simulink model "positionloop"  (R2024a)
settings: Solver=FixedStepAuto  StartTime=0.0  StopTime=5  FixedStep=1e-4  RelTol=1e-3
undefined symbols (not defined in the file): curr_d_ki, curr_d_kp, curr_q_ki, curr_q_kp, Ke, Kt, Pn, spd_ki, spd_kp, Udc
libraries: slpidlib x12, simulink x7, mcbplantlib x2, autolibpmsmexterior x2
(part 1 of 2)
settings Model: DataDictionary=positionloop.sldd  VariantFading=off  Creator=Administrator  LastModifiedBy=WuHongrui
settings OptimizationCC: DefaultParameterBehavior=Inlined  UseDivisionForNetSlopeComputation=on  GainParamInheritBuiltInType=on  UseFloatMulNetSlope=on  InlineInvariantSignals=on  PassReuseOutputArgsAs=Individual arguments  ZeroExternalMemoryAtStartup=off  ZeroInternalMemoryAtStartup=off  NoFixptDivByZeroProtection=on  EfficientFloat2IntCast=on  LifeSpan=1  OptimizeBlockOrder=speed  DifferentSizesBufferReuse=on  EfficientTunableParamExpr=on
settings DebuggingCC: ParameterTunabilityLossMsg=error  UnconnectedInputMsg=warning  UnconnectedOutputMsg=warning  UnconnectedLineMsg=warning
settings HardwareCC: ProdBitPerPointer=32  ProdBitPerSizeT=32  ProdBitPerPtrDiffT=32  ProdLargestAtomicInteger=Long  ProdLargestAtomicFloat=Double  ProdWordSize=32  ProdLongLongMode=on  ProdHWDeviceType=ARM Compatible->ARM Cortex-M
settings ModelReferenceCC: EnableRefExpFcnMdlSchedulingChecks=on
settings SFSimCC: MATLABDynamicMemAlloc=off
settings RTWCC: Description=Embedded Coder  SystemTargetFile=ert.tlc  GenCodeOnly=on  TemplateMakefile=ert_default_tmf  GenerateReport=on  LaunchReport=on  GenerateCodeReplacementReport=on  GPUComputeCapability=3.5  DLArmComputeVersion=19.05
settings CodeAppCC: ForceParamTrailComments=on  IgnoreCustomStorageClasses=off  OperatorAnnotations=on  SimulinkDataObjDesc=on  SFDataObjDesc=on  CustomSymbolStrGlobalVar=rt$N$M  CustomSymbolStrType=$N$M  CustomSymbolStrFcn=$N$M$F  CustomSymbolStrMacro=$N$M  InsertBlockDesc=on
settings ERTTargetCC: TargetLangStandard=C99 (ISO)  CodeReplacementLibrary=ARM Cortex-M  IncludeMdlTerminateFcn=off  CombineSignalStateStructs=on  SuppressErrorStatus=on  SupportAbsoluteTime=off  SupportComplex=off  InlinedParameterPlacement=NonHierarchical  ERTCustomFileTemplate=example_file_process.tlc  ERTFilePackagingFormat=CompactWithDataFile

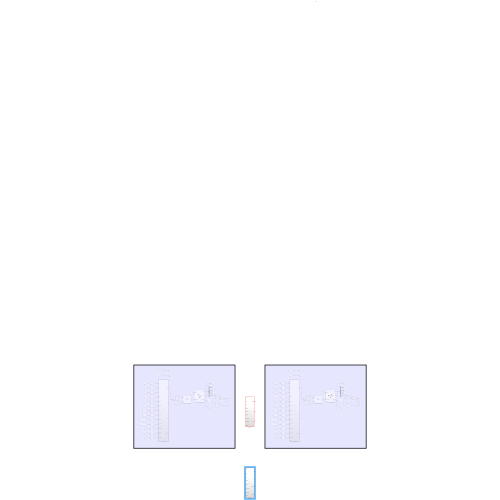
[thumbnail: Simulink's stored preview of the top-level diagram]
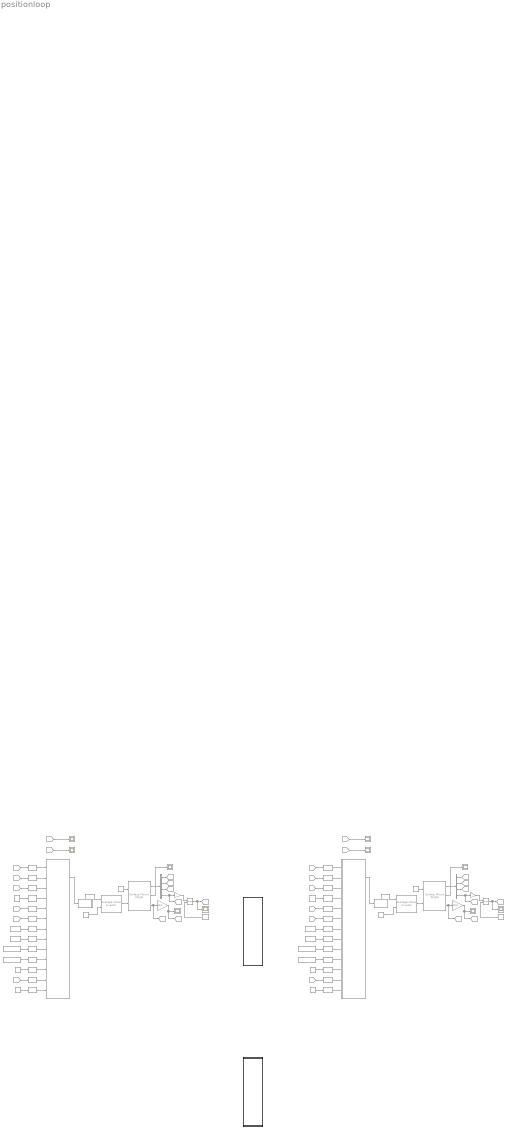
== system positionloop ==
  note: rad
  note: rad/s
  note: rpm
  note: rpm
  note: rad/s
  note: rpm
  note: rpm
  Average-Value Inverter3 : mcbplantlib/Average-Value Inverter  Commented=on
  Average-Value Inverter4 : mcbplantlib/Average-Value Inverter  Commented=on
  Bus Selector3 : BusSelector  Commented=on  OutputSignals=IaStator,IbStator,IcStator,MtrPos
  Bus Selector4 : BusSelector  Commented=on  OutputSignals=IaStator,IbStator,IcStator,MtrPos
  Constant26 : Constant  Commented=on  Value=0
  Constant28 : Constant  Commented=on  Value=0.515264878487547
  Constant34 : Constant  Commented=on  Value=pi/2
  Constant35 : Constant  Commented=on  Value=2*pi  OutDataTypeStr=single
  Constant36 : Constant  Commented=on  Value=0.003389
  Constant37 : Constant  Commented=on  Value=0.00144
  Constant38 : Constant  Commented=on  Value=Udc
  Constant39 : Constant  Commented=on  Value=Udc  OutDataTypeStr=single
  Constant40 : Constant  Commented=on  Value=987.649638453674
  Constant41 : Constant  Commented=on  Value=5
  Constant42 : Constant  Commented=on  Value=0
  Constant43 : Constant  Commented=on  Value=0.515264878487547
  Constant44 : Constant  Commented=on  Value=pi/2
  Constant45 : Constant  Commented=on  Value=2*pi  OutDataTypeStr=single
  Constant46 : Constant  Commented=on  Value=0.003389
  Constant47 : Constant  Commented=on  Value=0.00144
  Constant48 : Constant  Commented=on  Value=Udc
  Constant49 : Constant  Commented=on  Value=Udc  OutDataTypeStr=single
  Constant50 : Constant  Commented=on  Value=987.649638453674
  Constant51 : Constant  Commented=on  Value=5
  Data Type Conversion{35..60} (26 alike) : DataTypeConversion  Commented=on  OutDataTypeStr=single  SaturateOnIntegerOverflow=off  RndMeth=Floor
  From21 : From  Commented=on  GotoTag=ib
  From22 : From  Commented=on  GotoTag=ic
  From23 : From  Commented=on  GotoTag=W
  From24 : From  Commented=on  GotoTag=ia
  From25 : From  Commented=on  GotoTag=theta_e  TagVisibility=global
  From26 : From  Commented=on  GotoTag=Wrpm
  From{27..28,35..36} (4 alike) : From  Commented=on  GotoTag=theta  TagVisibility=global
  From29 : From  Commented=on  GotoTag=ib
  From30 : From  Commented=on  GotoTag=ic
  From31 : From  Commented=on  GotoTag=W
  From32 : From  Commented=on  GotoTag=ia
  From33 : From  Commented=on  GotoTag=theta_e  TagVisibility=global
  From34 : From  Commented=on  GotoTag=Wrpm
  Gain10 : Gain  Commented=on  Gain=Pn  OutDataTypeStr=single
  Gain7 : Gain  Commented=on  Gain=30/pi  OutDataTypeStr=single
  Gain8 : Gain  Commented=on  Gain=Pn  OutDataTypeStr=single
  Gain9 : Gain  Commented=on  Gain=30/pi  OutDataTypeStr=single
  Goto21 : Goto  Commented=on  GotoTag=ib
  Goto22 : Goto  Commented=on  GotoTag=ic
  Goto23 : Goto  Commented=on  GotoTag=theta_e  TagVisibility=global
  Goto24 : Goto  Commented=on  GotoTag=Wrpm
  Goto25 : Goto  Commented=on  GotoTag=W
  Goto26 : Goto  Commented=on  GotoTag=theta  TagVisibility=global
  Goto27 : Goto  Commented=on  GotoTag=ia
  Goto28 : Goto  Commented=on  GotoTag=ib
  Goto29 : Goto  Commented=on  GotoTag=ic
  Goto30 : Goto  Commented=on  GotoTag=theta_e  TagVisibility=global
  Goto31 : Goto  Commented=on  GotoTag=Wrpm
  Goto32 : Goto  Commented=on  GotoTag=W
  Goto33 : Goto  Commented=on  GotoTag=theta  TagVisibility=global
  Goto34 : Goto  Commented=on  GotoTag=ia
  Mod4 : Math  Commented=on  Operator=mod  OutputSignalType=real
  Mod5 : Math  Commented=on  Operator=mod  OutputSignalType=real
  Scope{17..26} (10 alike) : Scope  Commented=on
  Subsystem3 : Subsystem  Commented=on
      settings: PortSchema="{\"entries\":[{\"content\":{\"sides\":[{\"content\":{\"connectorIds\":[\"In1\"]},\"type\":\"ConnectorPlacement.EquallySpacedRectSide\",\"uuid\":\"8ccc51de-fa2a-4900-80a3-4cdf9aa76f01\"},{\"content\":{\"connectorIds\":[],\"side\":\"RIGHT\"},\"type\":\"ConnectorPlacement.EquallySpacedRectSide\",\"uuid\":\"32c06e0d-3f1d-4948-af96-e310e54308a0\"},{\"content\":{\"connectorIds\":[\"Out1\"],\"side\":\"TOP\"},\"type\":\"ConnectorPlacement.EquallySpacedRectSide\",\"uuid\":\"a9066067-2c54-42a8-b4d7-fb86ac71b860\"}]},\"type\":\"ConnectorPlacement.EquallySpacedConnector\",\"uuid\":\"e4576975-acad-4e16-822f-2c2e7f23d7a7\"}],\"packageUris\":[\"http://schema.mathworks.com/mf0/Connector/R2020b\"],\"version\":\"1.0\"}"
  Subsystem4 : Subsystem  Commented=on
      settings: PortSchema="{\"entries\":[{\"content\":{\"sides\":[{\"content\":{\"connectorIds\":[\"In1\"]},\"type\":\"ConnectorPlacement.EquallySpacedRectSide\",\"uuid\":\"8ccc51de-fa2a-4900-80a3-4cdf9aa76f01\"},{\"content\":{\"connectorIds\":[],\"side\":\"RIGHT\"},\"type\":\"ConnectorPlacement.EquallySpacedRectSide\",\"uuid\":\"32c06e0d-3f1d-4948-af96-e310e54308a0\"},{\"content\":{\"connectorIds\":[\"Out1\"],\"side\":\"TOP\"},\"type\":\"ConnectorPlacement.EquallySpacedRectSide\",\"uuid\":\"a9066067-2c54-42a8-b4d7-fb86ac71b860\"}]},\"type\":\"ConnectorPlacement.EquallySpacedConnector\",\"uuid\":\"e4576975-acad-4e16-822f-2c2e7f23d7a7\"}],\"packageUris\":[\"http://schema.mathworks.com/mf0/Connector/R2020b\"],\"version\":\"1.0\"}"
  Surface Mount PMSM3 : autolibpmsmexterior/Surface Mount PMSM  Commented=on  port_config=Torque  sim_type=Discrete  Ts=1e-4  P=Pn  Rs=Rs  Ldq_=L  KConstText=Torque constant (Kt):  lambda_pm=flux  Ke=0.0059268  Kt=Kt  mechanical=[0.096e-4, 2e-5, 0]  idq0=[0 0]  theta_init=0  omega_init=0  KConst=Kt  lambda_pm_calc=0.011  RefBlkName='autolibpmsmexterior/Surface Mount PMSM'  aMode=5  Ldq="[0.0017      0.0017]"
  Surface Mount PMSM4 : autolibpmsmexterior/Surface Mount PMSM  Commented=on  port_config=Torque  sim_type=Discrete  Ts=1e-4  P=Pn  Rs=Rs  Ldq_=L  KConstText=Torque constant (Kt):  lambda_pm=flux  Ke=0.0059268  Kt=Kt  mechanical=[0.096e-4, 2e-5, 0]  idq0=[0 0]  theta_init=0  omega_init=0  KConst=Kt  lambda_pm_calc=0.011  RefBlkName='autolibpmsmexterior/Surface Mount PMSM'  aMode=5  Ldq="[0.0017      0.0017]"
  currloop : Subsystem  TreatAsAtomicUnit=on
  currloop1 : Subsystem  TreatAsAtomicUnit=on
  triloop_feedforward : Subsystem  Commented=on  TreatAsAtomicUnit=on
  triloop_tune : Subsystem  Commented=on  TreatAsAtomicUnit=on
  wires:
  Surface Mount PMSM3/3 -> Gain7/1, Goto25/1
  Data Type Conversion42/1 -> triloop_tune/6(SpeedFd)
  triloop_tune/1(tABC) -> Subsystem3/1(DutyIn)
  Data Type Conversion36/1 -> triloop_tune/2(ib)
  Surface Mount PMSM3/1 -> Bus Selector3/1
  Bus Selector3/3 -> Goto22/1  "<IcStator>"
  Bus Selector3/4 -> Goto26/1, Gain8/1  "<MtrPos>"
  Subsystem3/1(DutyOut) -> Average-Value Inverter3/1
  Average-Value Inverter3/1 -> Surface Mount PMSM3/2
  From24/1 -> Data Type Conversion35/1
  Bus Selector3/2 -> Goto21/1  "<IbStator>"
  Constant35/1 -> Mod4/2
  Constant38/1 -> Average-Value Inverter3/2
  Mod4/1 -> Scope19/1, Goto23/1
  From22/1 -> Data Type Conversion38/1
  Bus Selector3/1 -> Goto27/1  "<IaStator>"
  Constant36/1 -> Data Type Conversion43/1
  From21/1 -> Data Type Conversion36/1
  Constant28/1 -> Data Type Conversion45/1
  Data Type Conversion44/1 -> triloop_tune/8(I_speed)
  From25/1 -> Data Type Conversion41/1
  Data Type Conversion45/1 -> triloop_tune/9(P_current)
  From23/1 -> Data Type Conversion42/1
  Data Type Conversion43/1 -> triloop_tune/7(P_speed)
  Data Type Conversion41/1 -> triloop_tune/5(theta_e)
  Gain8/1 -> Mod4/1
  Data Type Conversion39/1 -> triloop_tune/4(VBUS)
  Surface Mount PMSM3/2 -> Scope18/1  "Iab_fb"
  Data Type Conversion35/1 -> triloop_tune/1(ia)
  From26/1 -> Scope20/1
  Gain7/1 -> Scope17/1, Goto24/1
  Constant26/1 -> Surface Mount PMSM3/1
  Constant39/1 -> Data Type Conversion39/1
  Data Type Conversion38/1 -> triloop_tune/3(ic)
  Data Type Conversion37/1 -> triloop_tune/10(I_current)
  Constant40/1 -> Data Type Conversion37/1
  Constant37/1 -> Data Type Conversion44/1
  Data Type Conversion47/1 -> triloop_tune/13(P_position)
  Data Type Conversion46/1 -> triloop_tune/12(PositionFd)
  Data Type Conversion40/1 -> triloop_tune/11(PositionRef)
  Constant34/1 -> Data Type Conversion40/1
  From27/1 -> Data Type Conversion46/1
  Constant41/1 -> Data Type Conversion47/1
  From28/1 -> Scope21/1
  Data Type Conversion53/1 -> triloop_feedforward/11(PositionRef)
  Constant51/1 -> Data Type Conversion60/1
  Constant42/1 -> Surface Mount PMSM4/1
  From34/1 -> Scope25/1
  From31/1 -> Data Type Conversion55/1
  Data Type Conversion60/1 -> triloop_feedforward/13(P_position)
  Data Type Conversion57/1 -> triloop_feedforward/8(I_speed)
  Data Type Conversion58/1 -> triloop_feedforward/9(P_current)
  Data Type Conversion54/1 -> triloop_feedforward/5(theta_e)
  Data Type Conversion48/1 -> triloop_feedforward/1(ia)
  Surface Mount PMSM4/2 -> Scope23/1  "Iab_fb"
  Gain10/1 -> Mod5/1
  Data Type Conversion59/1 -> triloop_feedforward/12(PositionFd)
  Constant43/1 -> Data Type Conversion58/1
  Data Type Conversion52/1 -> triloop_feedforward/4(VBUS)
  Data Type Conversion56/1 -> triloop_feedforward/7(P_speed)
  From30/1 -> Data Type Conversion51/1
  From29/1 -> Data Type Conversion49/1
  Gain9/1 -> Scope22/1, Goto31/1
  Constant48/1 -> Average-Value Inverter4/2
  Constant46/1 -> Data Type Conversion56/1
  Mod5/1 -> Scope24/1, Goto30/1
  Bus Selector4/3 -> Goto29/1  "<IcStator>"
  Bus Selector4/2 -> Goto28/1  "<IbStator>"
  Data Type Conversion49/1 -> triloop_feedforward/2(ib)
  Bus Selector4/4 -> Goto33/1, Gain10/1  "<MtrPos>"
  Constant45/1 -> Mod5/2
  Average-Value Inverter4/1 -> Surface Mount PMSM4/2
  Surface Mount PMSM4/1 -> Bus Selector4/1
  Subsystem4/1(DutyOut) -> Average-Value Inverter4/1
  Surface Mount PMSM4/3 -> Gain9/1, Goto32/1
  From33/1 -> Data Type Conversion54/1
  From32/1 -> Data Type Conversion48/1
  triloop_feedforward/1(tABC) -> Subsystem4/1(DutyIn)
  Data Type Conversion55/1 -> triloop_feedforward/6(SpeedFd)
  Data Type Conversion51/1 -> triloop_feedforward/3(ic)
  Constant50/1 -> Data Type Conversion50/1
  Constant49/1 -> Data Type Conversion52/1
  Constant47/1 -> Data Type Conversion57/1
  Constant44/1 -> Data Type Conversion53/1
  Data Type Conversion50/1 -> triloop_feedforward/10(I_current)
  Bus Selector4/1 -> Goto34/1  "<IaStator>"
  From35/1 -> Data Type Conversion59/1
  From36/1 -> Scope26/1

== system positionloop/Subsystem3 ==
  DutyIn : Inport
  Constant : Constant  Value=0.5  SampleTime=-1
  Gain : Gain  Gain=1/8000  ParamDataTypeStr=single
  Gain1 : Gain  Gain=-1
  Sum : Sum  Inputs=|+-
  Sum1 : Sum  Inputs=|++
  DutyOut : Outport
  wires:
  Sum/1 -> Gain1/1
  Constant/1 -> Sum1/2, Sum/2
  DutyIn/1 -> Gain/1
  Gain1/1 -> Sum1/1
  Sum1/1 -> DutyOut/1
  Gain/1 -> Sum/1

== system positionloop/Subsystem4 ==
  DutyIn : Inport
  Constant : Constant  Value=0.5  SampleTime=-1
  Gain : Gain  Gain=1/8000  ParamDataTypeStr=single
  Gain1 : Gain  Gain=-1
  Sum : Sum  Inputs=|+-
  Sum1 : Sum  Inputs=|++
  DutyOut : Outport
  wires:
  Sum/1 -> Gain1/1
  Constant/1 -> Sum1/2, Sum/2
  DutyIn/1 -> Gain/1
  Gain1/1 -> Sum1/1
  Sum1/1 -> DutyOut/1
  Gain/1 -> Sum/1

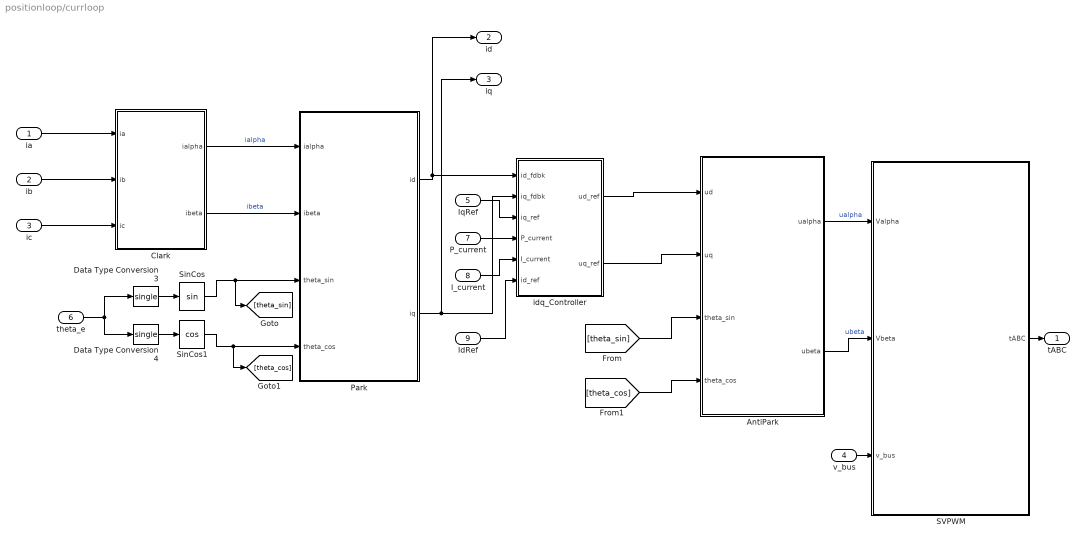
== system positionloop/currloop ==
  ia : Inport
  ib : Inport  Port=2
  ic : Inport  Port=3
  v_bus : Inport  Port=4
  IqRef : Inport  Port=5
  theta_e : Inport  Port=6
  P_current : Inport  Port=7
  I_current : Inport  Port=8
  IdRef : Inport  Port=9
  AntiPark : Subsystem
  Clark : Subsystem
  Data Type Conversion3 : DataTypeConversion  OutDataTypeStr=single  SaturateOnIntegerOverflow=off  RndMeth=Floor
  Data Type Conversion4 : DataTypeConversion  OutDataTypeStr=single  SaturateOnIntegerOverflow=off  RndMeth=Floor
  Park : Subsystem
  SVPWM : Subsystem  TreatAsAtomicUnit=on
  SinCos : Trigonometry
  SinCos1 : Trigonometry  Operator=cos
  idq_Controller : Subsystem
  tABC : Outport
  id : Outport  Port=2
  iq : Outport  Port=3
  wires:
  Data Type Conversion4/1 -> SinCos1/1
  Data Type Conversion3/1 -> SinCos/1
  AntiPark/2(ubeta) -> SVPWM/2(Vbeta)  "ubeta"
  AntiPark/1(ualpha) -> SVPWM/1(Valpha)  "ualpha"
  [theta_cos] -> AntiPark/4(theta_cos)
  [theta_sin] -> AntiPark/3(theta_sin)
  SinCos/1 -> Park/3(theta_sin), [theta_sin]
  theta_e/1 -> Data Type Conversion3/1, Data Type Conversion4/1
  SinCos1/1 -> Park/4(theta_cos), [theta_cos]
  v_bus/1 -> SVPWM/3(v_bus)
  SVPWM/1(tABC) -> tABC/1
  ib/1 -> Clark/2(ib)
  ia/1 -> Clark/1(ia)
  ic/1 -> Clark/3(ic)
  Clark/1(ialpha) -> Park/1(ialpha)  "ialpha"
  Clark/2(ibeta) -> Park/2(ibeta)  "ibeta"
  idq_Controller/1(ud_ref) -> AntiPark/1(ud)
  idq_Controller/2(uq_ref) -> AntiPark/2(uq)
  Park/1(id) -> id/1, idq_Controller/1(id_fdbk)
  Park/2(iq) -> iq/1, idq_Controller/2(iq_fdbk)
  IqRef/1 -> idq_Controller/3(iq_ref)
  I_current/1 -> idq_Controller/5(I_current)
  P_current/1 -> idq_Controller/4(P_current)
  IdRef/1 -> idq_Controller/6(id_ref)

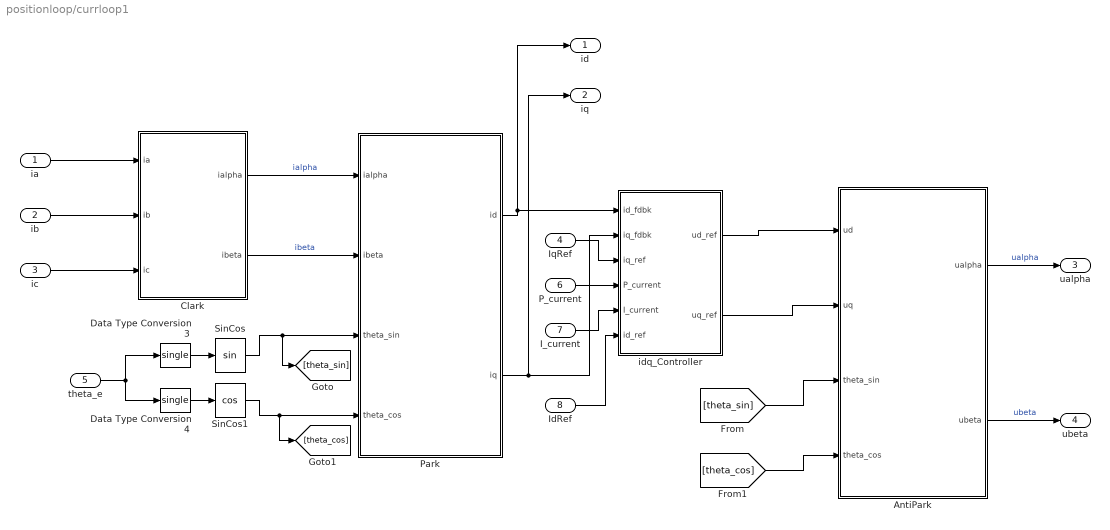
== system positionloop/currloop1 ==
  ia : Inport
  ib : Inport  Port=2
  ic : Inport  Port=3
  IqRef : Inport  Port=4
  theta_e : Inport  Port=5
  P_current : Inport  Port=6
  I_current : Inport  Port=7
  IdRef : Inport  Port=8
  AntiPark : Subsystem
  Clark : Subsystem
  Data Type Conversion3 : DataTypeConversion  OutDataTypeStr=single  SaturateOnIntegerOverflow=off  RndMeth=Floor
  Data Type Conversion4 : DataTypeConversion  OutDataTypeStr=single  SaturateOnIntegerOverflow=off  RndMeth=Floor
  Park : Subsystem
  SinCos : Trigonometry
  SinCos1 : Trigonometry  Operator=cos
  idq_Controller : Subsystem
  id : Outport
  iq : Outport  Port=2
  ualpha : Outport  Port=3
  ubeta : Outport  Port=4
  wires:
  Data Type Conversion4/1 -> SinCos1/1
  Data Type Conversion3/1 -> SinCos/1
  [theta_cos] -> AntiPark/4(theta_cos)
  [theta_sin] -> AntiPark/3(theta_sin)
  SinCos/1 -> Park/3(theta_sin), [theta_sin]
  theta_e/1 -> Data Type Conversion3/1, Data Type Conversion4/1
  SinCos1/1 -> Park/4(theta_cos), [theta_cos]
  ib/1 -> Clark/2(ib)
  ia/1 -> Clark/1(ia)
  ic/1 -> Clark/3(ic)
  Clark/1(ialpha) -> Park/1(ialpha)  "ialpha"
  Clark/2(ibeta) -> Park/2(ibeta)  "ibeta"
  idq_Controller/1(ud_ref) -> AntiPark/1(ud)
  idq_Controller/2(uq_ref) -> AntiPark/2(uq)
  Park/1(id) -> id/1, idq_Controller/1(id_fdbk)
  Park/2(iq) -> iq/1, idq_Controller/2(iq_fdbk)
  IqRef/1 -> idq_Controller/3(iq_ref)
  I_current/1 -> idq_Controller/5(I_current)
  P_current/1 -> idq_Controller/4(P_current)
  IdRef/1 -> idq_Controller/6(id_ref)
  AntiPark/1(ualpha) -> ualpha/1  "ualpha"
  AntiPark/2(ubeta) -> ubeta/1  "ubeta"

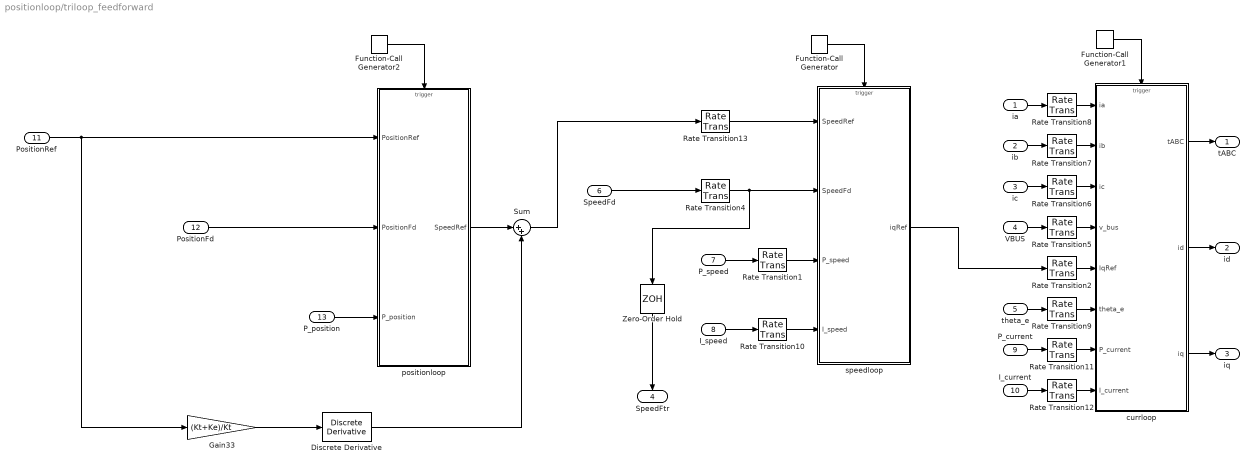
== system positionloop/triloop_feedforward ==
  ia : Inport
  ib : Inport  Port=2
  ic : Inport  Port=3
  VBUS : Inport  Port=4
  theta_e : Inport  Port=5
  SpeedFd : Inport  Port=6
  P_speed : Inport  Port=7
  I_speed : Inport  Port=8
  P_current : Inport  Port=9
  I_current : Inport  Port=10
  PositionRef : Inport  Port=11
  PositionFd : Inport  Port=12
  P_position : Inport  Port=13
  Discrete Derivative : simulink/Discrete/Discrete Derivative  gainval=0.35  ICPrevScaledInput=0.0  OutMin=[]  OutMax=[]  OutDataType=fixdt(1, 16)  OutScaling=2^-10  DoSatur=off
  Function-Call Generator : simulink/Ports & Subsystems/Function-Call Generator  sample_time=1e-3  numberOfIterations=1  DisallowWideOutput=off
  Function-Call Generator1 : simulink/Ports & Subsystems/Function-Call Generator  sample_time=1e-4  numberOfIterations=1  DisallowWideOutput=off
  Function-Call Generator2 : simulink/Ports & Subsystems/Function-Call Generator  sample_time=1e-2  numberOfIterations=1  DisallowWideOutput=off
  Gain33 : Gain  Gain=(Kt+Ke)/Kt
  Rate Transition{1..2,4..13} (12 alike) : RateTransition
  Sum : Sum  Inputs=|++
  Zero-Order Hold : ZeroOrderHold  SampleTime=-1
  currloop : Subsystem  TreatAsAtomicUnit=on
  positionloop : Subsystem
  speedloop : Subsystem
  tABC : Outport
  id : Outport  Port=2
  iq : Outport  Port=3
  SpeedFtr : Outport  Port=4
  wires:
  currloop/1(tABC) -> tABC/1
  VBUS/1 -> Rate Transition5/1
  ib/1 -> Rate Transition7/1
  ia/1 -> Rate Transition8/1
  ic/1 -> Rate Transition6/1
  Function-Call Generator/1 -> speedloop/Trigger
  Rate Transition13/1 -> speedloop/1(SpeedRef)
  theta_e/1 -> Rate Transition9/1
  Rate Transition2/1 -> currloop/5(IqRef)
  Rate Transition5/1 -> currloop/4(v_bus)
  Rate Transition6/1 -> currloop/3(ic)
  Rate Transition7/1 -> currloop/2(ib)
  Rate Transition8/1 -> currloop/1(ia)
  Rate Transition9/1 -> currloop/6(theta_e)
  Rate Transition4/1 -> speedloop/2(SpeedFd), Zero-Order Hold/1
  SpeedFd/1 -> Rate Transition4/1
  Function-Call Generator1/1 -> currloop/Trigger
  P_speed/1 -> Rate Transition1/1
  I_speed/1 -> Rate Transition10/1
  P_current/1 -> Rate Transition11/1
  I_current/1 -> Rate Transition12/1
  speedloop/1(iqRef) -> Rate Transition2/1
  Rate Transition1/1 -> speedloop/3(P_speed)
  Rate Transition10/1 -> speedloop/4(I_speed)
  Rate Transition11/1 -> currloop/7(P_current)
  Rate Transition12/1 -> currloop/8(I_current)
  currloop/3(iq) -> iq/1
  currloop/2(id) -> id/1
  Zero-Order Hold/1 -> SpeedFtr/1
  PositionFd/1 -> positionloop/2(PositionFd)
  P_position/1 -> positionloop/3(P_position)
  Function-Call Generator2/1 -> positionloop/Trigger
  Gain33/1 -> Discrete Derivative/1
  Sum/1 -> Rate Transition13/1
  positionloop/1(SpeedRef) -> Sum/1
  PositionRef/1 -> Gain33/1, positionloop/1(PositionRef)
  Discrete Derivative/1 -> Sum/2

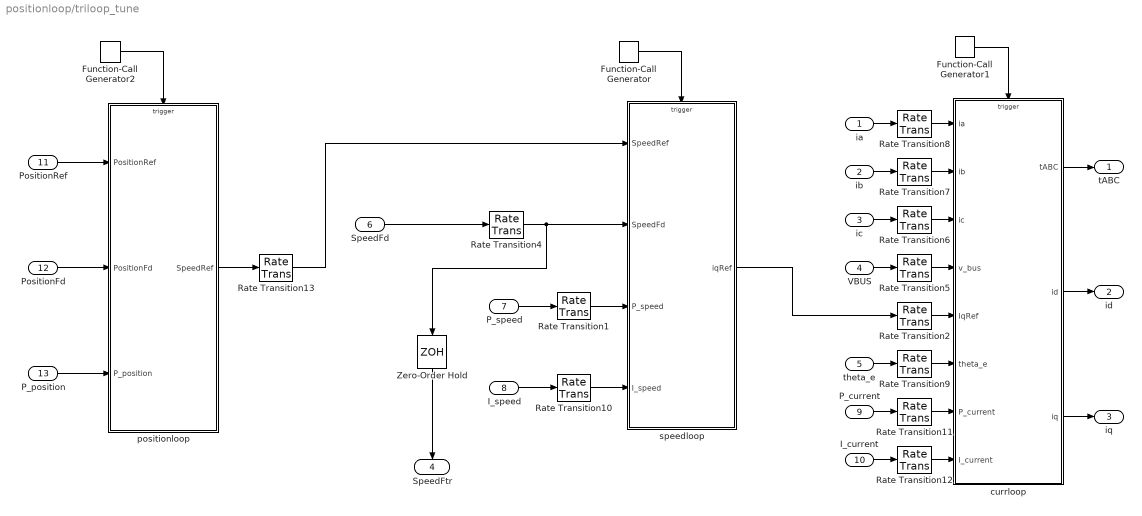
== system positionloop/triloop_tune ==
  ia : Inport
  ib : Inport  Port=2
  ic : Inport  Port=3
  VBUS : Inport  Port=4
  theta_e : Inport  Port=5
  SpeedFd : Inport  Port=6
  P_speed : Inport  Port=7
  I_speed : Inport  Port=8
  P_current : Inport  Port=9
  I_current : Inport  Port=10
  PositionRef : Inport  Port=11
  PositionFd : Inport  Port=12
  P_position : Inport  Port=13
  Function-Call Generator : simulink/Ports & Subsystems/Function-Call Generator  sample_time=1e-3  numberOfIterations=1  DisallowWideOutput=off
  Function-Call Generator1 : simulink/Ports & Subsystems/Function-Call Generator  sample_time=1e-4  numberOfIterations=1  DisallowWideOutput=off
  Function-Call Generator2 : simulink/Ports & Subsystems/Function-Call Generator  sample_time=1e-3  numberOfIterations=1  DisallowWideOutput=off
  Rate Transition{1..2,4..13} (12 alike) : RateTransition
  Zero-Order Hold : ZeroOrderHold  SampleTime=-1
  currloop : Subsystem  TreatAsAtomicUnit=on
  positionloop : Subsystem
  speedloop : Subsystem
  tABC : Outport
  id : Outport  Port=2
  iq : Outport  Port=3
  SpeedFtr : Outport  Port=4
  wires:
  currloop/1(tABC) -> tABC/1
  VBUS/1 -> Rate Transition5/1
  ib/1 -> Rate Transition7/1
  ia/1 -> Rate Transition8/1
  ic/1 -> Rate Transition6/1
  Function-Call Generator/1 -> speedloop/Trigger
  Rate Transition13/1 -> speedloop/1(SpeedRef)
  theta_e/1 -> Rate Transition9/1
  Rate Transition2/1 -> currloop/5(IqRef)
  Rate Transition5/1 -> currloop/4(v_bus)
  Rate Transition6/1 -> currloop/3(ic)
  Rate Transition7/1 -> currloop/2(ib)
  Rate Transition8/1 -> currloop/1(ia)
  Rate Transition9/1 -> currloop/6(theta_e)
  Rate Transition4/1 -> speedloop/2(SpeedFd), Zero-Order Hold/1
  SpeedFd/1 -> Rate Transition4/1
  Function-Call Generator1/1 -> currloop/Trigger
  P_speed/1 -> Rate Transition1/1
  I_speed/1 -> Rate Transition10/1
  P_current/1 -> Rate Transition11/1
  I_current/1 -> Rate Transition12/1
  speedloop/1(iqRef) -> Rate Transition2/1
  Rate Transition1/1 -> speedloop/3(P_speed)
  Rate Transition10/1 -> speedloop/4(I_speed)
  Rate Transition11/1 -> currloop/7(P_current)
  Rate Transition12/1 -> currloop/8(I_current)
  currloop/3(iq) -> iq/1
  currloop/2(id) -> id/1
  Zero-Order Hold/1 -> SpeedFtr/1
  positionloop/1(SpeedRef) -> Rate Transition13/1
  PositionRef/1 -> positionloop/1(PositionRef)
  PositionFd/1 -> positionloop/2(PositionFd)
  P_position/1 -> positionloop/3(P_position)
  Function-Call Generator2/1 -> positionloop/Trigger

== system positionloop/currloop/AntiPark ==
  note: Valpha = ud*cos(theta) - uq*sin(theta);
      | Vbeta = ud*sin(theta) + uq*cos(theta);
  ud : Inport
  uq : Inport  Port=2
  theta_sin : Inport  Port=3
  theta_cos : Inport  Port=4
  Add : Sum  Inputs=+-
  Add1 : Sum
  Product{,1..3} (4 alike) : Product
  ualpha : Outport  OutDataTypeStr=single
  ubeta : Outport  Port=2  OutDataTypeStr=single
  wires:
  Product2/1 -> Add1/1
  Product/1 -> Add/1
  Add/1 -> ualpha/1
  Product3/1 -> Add1/2
  ud/1 -> Product/1, Product2/1
  theta_sin/1 -> Product1/2, Product2/2
  theta_cos/1 -> Product3/2, Product/2
  uq/1 -> Product1/1, Product3/1
  Product1/1 -> Add/2
  Add1/1 -> ubeta/1

== system positionloop/currloop/Clark ==
  note: ialpha = ia*2/3-(ib+ic)/3;
      | ibeta = (ib-ic)*sqrt(3)/3;
  ia : Inport  OutDataTypeStr=single
  ib : Inport  Port=2  OutDataTypeStr=single
  ic : Inport  Port=3  OutDataTypeStr=single
  Add : Sum  OutDataTypeStr=single  AccumDataTypeStr=single
  Add1 : Sum  Inputs=+-  OutDataTypeStr=single  AccumDataTypeStr=single
  Add2 : Sum  Inputs=+-  OutDataTypeStr=single  AccumDataTypeStr=single
  Gain : Gain  Gain=2/3  ParamDataTypeStr=single
  Gain1 : Gain  Gain=1/3  ParamDataTypeStr=single
  Gain2 : Gain  Gain=sqrt(3)/3  ParamDataTypeStr=single
  ialpha : Outport  OutDataTypeStr=single
  ibeta : Outport  Port=2  OutDataTypeStr=single
  wires:
  Add1/1 -> ialpha/1
  ia/1 -> Gain/1
  Gain2/1 -> ibeta/1
  ib/1 -> Add/1, Add2/1
  Gain/1 -> Add1/1
  Add2/1 -> Gain2/1
  Add/1 -> Gain1/1
  ic/1 -> Add/2, Add2/2
  Gain1/1 -> Add1/2

== system positionloop/currloop/Park ==
  note: id = ialpha*cos(theta)+ibeta*sin(theta);
      | iq = -ialpha*sin(theta)+ibeta*cos(theta);
  ialpha : Inport  OutDataTypeStr=single
  ibeta : Inport  Port=2  OutDataTypeStr=single
  theta_sin : Inport  Port=3  OutDataTypeStr=single
  theta_cos : Inport  Port=4  OutDataTypeStr=single
  Add : Sum  OutDataTypeStr=single  AccumDataTypeStr=single
  Add1 : Sum  Inputs=-+  OutDataTypeStr=single  AccumDataTypeStr=single
  Product{,1..3} (4 alike) : Product  OutDataTypeStr=single
  id : Outport  OutDataTypeStr=single
  iq : Outport  Port=2  OutDataTypeStr=single
  wires:
  theta_cos/1 -> Product/2, Product3/2
  ibeta/1 -> Product1/1, Product3/1
  Product1/1 -> Add/2
  Add1/1 -> iq/1
  Add/1 -> id/1
  Product3/1 -> Add1/2
  ialpha/1 -> Product/1, Product2/1
  Product2/1 -> Add1/1
  Product/1 -> Add/1
  theta_sin/1 -> Product1/2, Product2/2

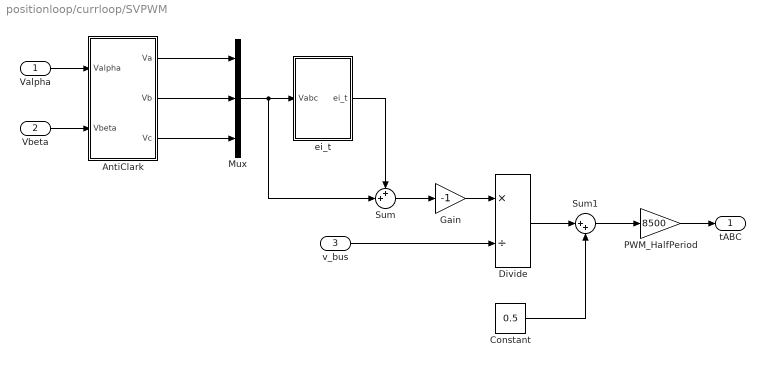
== system positionloop/currloop/SVPWM ==
  Valpha : Inport  OutDataTypeStr=single
  Vbeta : Inport  Port=2  OutDataTypeStr=single
  v_bus : Inport  Port=3  OutDataTypeStr=single
  AntiClark : Subsystem
  Constant : Constant  Value=0.5  OutDataTypeStr=single
  Divide : Product  Inputs=*/  OutDataTypeStr=single
  Gain : Gain  Gain=-1  OutDataTypeStr=single
  Mux : Mux  Inputs=3
  PWM_HalfPeriod : Gain  Gain=8500  OutDataTypeStr=single
  Sum : Sum  Inputs=++|  OutDataTypeStr=single
  Sum1 : Sum  Inputs=|++  OutDataTypeStr=single
  ei_t : Subsystem
  tABC : Outport  OutDataTypeStr=single
  wires:
  Gain/1 -> Divide/1
  v_bus/1 -> Divide/2
  PWM_HalfPeriod/1 -> tABC/1
  Sum1/1 -> PWM_HalfPeriod/1
  Constant/1 -> Sum1/2
  Divide/1 -> Sum1/1
  Mux/1 -> ei_t/1(Vabc), Sum/2
  Sum/1 -> Gain/1
  AntiClark/3(Vc) -> Mux/3
  AntiClark/2(Vb) -> Mux/2
  AntiClark/1(Va) -> Mux/1
  ei_t/1(ei_t) -> Sum/1
  Vbeta/1 -> AntiClark/2(Vbeta)
  Valpha/1 -> AntiClark/1(Valpha)

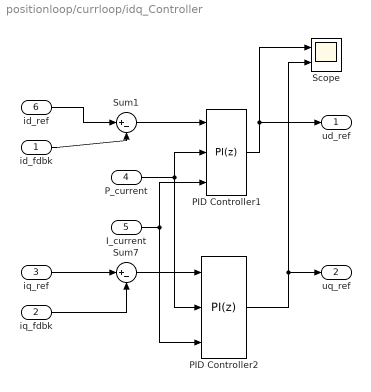
== system positionloop/currloop/idq_Controller ==
  id_fdbk : Inport  OutDataTypeStr=single
  iq_fdbk : Inport  Port=2  OutDataTypeStr=single
  iq_ref : Inport  Port=3  OutDataTypeStr=single
  P_current : Inport  Port=4  OutDataTypeStr=single
  I_current : Inport  Port=5  OutDataTypeStr=single
  id_ref : Inport  Port=6  OutDataTypeStr=single
  PID Controller1 : slpidlib/PID Controller  Controller=PI  Form=Parallel  TimeDomain=Discrete-time  UseExternalTs=off  SampleTime=-1  IntegratorMethod=Forward Euler  FilterMethod=Forward Euler  ControllerParametersSource=external  P=curr_d_kp  I=curr_d_ki  UseKiTs=off  D=0  UseExternalDerivativeSource=off  N=100  UseFilter=on  TunerSelectOption=Transfer Function Based (PID Tuner App)  InitialConditionSource=internal  InitialConditionForIntegrator=0  InitialConditionForFilter=0  DifferentiatorICPrevScaledInput=0  ExternalReset=none  TrackingMode=off  Kt=1  LimitOutput=on  SatLimitsSource=internal  UpperSaturationLimit=48*0.9/sqrt(3)  LowerSaturationLimit=-48*0.9/sqrt(3)  LinearizeAsGain=on  AntiWindupMode=clamping  Kb=1  LimitIntegrator=off  UpperIntegratorSaturationLimit=inf  LowerIntegratorSaturationLimit=-inf  PGainOutDataTypeStr=single  PProdOutDataTypeStr=single  POutMin=[]  POutMax=[]  IGainOutDataTypeStr=int16  IProdOutDataTypeStr=int16  IOutMin=[]  IOutMax=[]  DOutMin=[]  DOutMax=[]  NOutMin=[]  NOutMax=[]  SumOutDataTypeStr=single  SumOutMin=[]  SumOutMax=[]  SaturationOutDataTypeStr=single  SaturationOutMin=[]  SaturationOutMax=[]  PParamMin=[]  PParamMax=[]  IParamMin=[]  IParamMax=[]  DParamMin=[]  DParamMax=[]  NParamMin=[]  NParamMax=[]  KbParamMin=[]  KbParamMax=[]  KtParamMin=[]  KtParamMax=[]  KbOutMin=[]  KbOutMax=[]  KtOutMin=[]  KtOutMax=[]  IntegratorOutMin=[]  IntegratorOutMax=[]  FilterOutMin=[]  FilterOutMax=[]  SumI1OutMin=[]  SumI1OutMax=[]  SumI2OutMin=[]  SumI2OutMax=[]  SumI3OutMin=[]  SumI3OutMax=[]  SumI4OutMin=[]  SumI4OutMax=[]  SumDOutMin=[]  SumDOutMax=[]  DifferentiatorOutMin=[]  DifferentiatorOutMax=[]  FilterDiffOutCoefMin=[]  FilterDiffOutCoefMax=[]  ReciprocalOutMin=[]  ReciprocalOutMax=[]  SumDenOutMin=[]  SumDenOutMax=[]  SumNumOutMin=[]  SumNumOutMax=[]  DivideOutMin=[]  DivideOutMax=[]  UdiffTsProdOutMin=[]  UdiffTsProdOutMax=[]  NTsProdOutMin=[]  NTsProdOutMax=[]  UintegralTsProdOutMin=[]  UintegralTsProdOutMax=[]  UngainTsProdOutMin=[]  UngainTsProdOutMax=[]  ClampingZeroOutDataTypeStr=Inherit: Inherit via back propagation  ClampingZeroOutMin=[]  ClampingZeroOutMax=[]  FilterDenConstantOutDataTypeStr=Inherit: Inherit via back propagation  FilterDenConstantOutMin=[]  FilterDenConstantOutMax=[]  PCopyOutDataTypeStr=Inherit: Inherit via back propagation  PCopyOutMin=[]  PCopyOutMax=[]  NCopyOutDataTypeStr=Inherit: Inherit via back propagation  NCopyOutMin=[]  NCopyOutMax=[]  IntegratorContinuousStateAttributes=''  IntegratorStateMustResolveToSignalObject=off  IntegratorRTWStateStorageClass=Auto  FilterContinuousStateAttributes=''  FilterStateMustResolveToSignalObject=off  FilterRTWStateStorageClass=Auto  ParallelPVariant=ExternalParameters  IdealPVariant=Disabled  IVariant=ExternalParameters  DVariant=Disabled  IntegratorVariant=Discrete  SatVariant=Enabled  AWVariant=DiscClampingParallel  PCopyVariant=Disabled  TRVariant=Disabled  FdbkBlocksVariant=Forward  IdealPFdbkVariant=Disabled  SatFdbkVariant=Disabled  DerivativeFilterVariant=Disabled  NVariant=Disabled  NCopyVariant=Disabled_SignalSpec  FilterICVariant=Disabled  IntegratorICVariant=InternalICs  ExternalResetVariant=Disabled  TRSumVariant=Passthrough  SumFdbkVariant=Disabled  SumVariant=Sum_PI  TsampFilterVariant=InternalTs  TsampNgainVariant=Passthrough  TsampIntegralVariant=Disabled_SignalSpec  ExternalSaturationOutDataTypeStr=Inherit: Same as second input  DerivativeSourceVariant=Disabled
  PID Controller2 : slpidlib/PID Controller  Controller=PI  Form=Parallel  TimeDomain=Discrete-time  UseExternalTs=off  SampleTime=-1  IntegratorMethod=Forward Euler  FilterMethod=Forward Euler  ControllerParametersSource=external  P=curr_q_kp  I=curr_q_ki  UseKiTs=off  D=0  UseExternalDerivativeSource=off  N=100  UseFilter=on  TunerSelectOption=Transfer Function Based (PID Tuner App)  InitialConditionSource=internal  InitialConditionForIntegrator=0  InitialConditionForFilter=0  DifferentiatorICPrevScaledInput=0  ExternalReset=none  TrackingMode=off  Kt=1  LimitOutput=on  SatLimitsSource=internal  UpperSaturationLimit=48*0.9/sqrt(3)  LowerSaturationLimit=-48*0.9/sqrt(3)  LinearizeAsGain=on  AntiWindupMode=clamping  Kb=1  LimitIntegrator=off  UpperIntegratorSaturationLimit=inf  LowerIntegratorSaturationLimit=-inf  PGainOutDataTypeStr=single  PProdOutDataTypeStr=single  POutMin=[]  POutMax=[]  IGainOutDataTypeStr=single  IProdOutDataTypeStr=single  IOutMin=[]  IOutMax=[]  DOutMin=[]  DOutMax=[]  NOutMin=[]  NOutMax=[]  SumOutDataTypeStr=single  SumOutMin=[]  SumOutMax=[]  SaturationOutDataTypeStr=single  SaturationOutMin=[]  SaturationOutMax=[]  PParamMin=[]  PParamMax=[]  IParamMin=[]  IParamMax=[]  DParamMin=[]  DParamMax=[]  NParamMin=[]  NParamMax=[]  KbParamMin=[]  KbParamMax=[]  KtParamMin=[]  KtParamMax=[]  KbOutMin=[]  KbOutMax=[]  KtOutMin=[]  KtOutMax=[]  IntegratorOutMin=[]  IntegratorOutMax=[]  FilterOutMin=[]  FilterOutMax=[]  SumI1OutMin=[]  SumI1OutMax=[]  SumI2OutMin=[]  SumI2OutMax=[]  SumI3OutMin=[]  SumI3OutMax=[]  SumI4OutMin=[]  SumI4OutMax=[]  SumDOutMin=[]  SumDOutMax=[]  DifferentiatorOutMin=[]  DifferentiatorOutMax=[]  FilterDiffOutCoefMin=[]  FilterDiffOutCoefMax=[]  ReciprocalOutMin=[]  ReciprocalOutMax=[]  SumDenOutMin=[]  SumDenOutMax=[]  SumNumOutMin=[]  SumNumOutMax=[]  DivideOutMin=[]  DivideOutMax=[]  UdiffTsProdOutMin=[]  UdiffTsProdOutMax=[]  NTsProdOutMin=[]  NTsProdOutMax=[]  UintegralTsProdOutMin=[]  UintegralTsProdOutMax=[]  UngainTsProdOutMin=[]  UngainTsProdOutMax=[]  ClampingZeroOutDataTypeStr=Inherit: Inherit via back propagation  ClampingZeroOutMin=[]  ClampingZeroOutMax=[]  FilterDenConstantOutDataTypeStr=Inherit: Inherit via back propagation  FilterDenConstantOutMin=[]  FilterDenConstantOutMax=[]  PCopyOutDataTypeStr=Inherit: Inherit via back propagation  PCopyOutMin=[]  PCopyOutMax=[]  NCopyOutDataTypeStr=Inherit: Inherit via back propagation  NCopyOutMin=[]  NCopyOutMax=[]  IntegratorContinuousStateAttributes=''  IntegratorStateMustResolveToSignalObject=off  IntegratorRTWStateStorageClass=Auto  FilterContinuousStateAttributes=''  FilterStateMustResolveToSignalObject=off  FilterRTWStateStorageClass=Auto  ParallelPVariant=ExternalParameters  IdealPVariant=Disabled  IVariant=ExternalParameters  DVariant=Disabled  IntegratorVariant=Discrete  SatVariant=Enabled  AWVariant=DiscClampingParallel  PCopyVariant=Disabled  TRVariant=Disabled  FdbkBlocksVariant=Forward  IdealPFdbkVariant=Disabled  SatFdbkVariant=Disabled  DerivativeFilterVariant=Disabled  NVariant=Disabled  NCopyVariant=Disabled_SignalSpec  FilterICVariant=Disabled  IntegratorICVariant=InternalICs  ExternalResetVariant=Disabled  TRSumVariant=Passthrough  SumFdbkVariant=Disabled  SumVariant=Sum_PI  TsampFilterVariant=InternalTs  TsampNgainVariant=Passthrough  TsampIntegralVariant=Disabled_SignalSpec  ExternalSaturationOutDataTypeStr=Inherit: Same as second input  DerivativeSourceVariant=Disabled
  Scope : Scope  NumInputPorts=2
  Sum1 : Sum  Inputs=|+-  OutDataTypeStr=single  AccumDataTypeStr=single
  Sum7 : Sum  Inputs=|+-  OutDataTypeStr=single  AccumDataTypeStr=single
  ud_ref : Outport  OutDataTypeStr=single
  uq_ref : Outport  Port=2  OutDataTypeStr=single
  wires:
  id_fdbk/1 -> Sum1/2
  id_ref/1 -> Sum1/1
  iq_fdbk/1 -> Sum7/2
  Sum1/1 -> PID Controller1/1
  Sum7/1 -> PID Controller2/1
  PID Controller1/1 -> Scope/1, ud_ref/1
  PID Controller2/1 -> Scope/2, uq_ref/1
  iq_ref/1 -> Sum7/1
  P_current/1 -> PID Controller2/2, PID Controller1/2
  I_current/1 -> PID Controller2/3, PID Controller1/3

== system positionloop/currloop1/AntiPark ==
  note: Valpha = ud*cos(theta) - uq*sin(theta);
      | Vbeta = ud*sin(theta) + uq*cos(theta);
  ud : Inport
  uq : Inport  Port=2
  theta_sin : Inport  Port=3
  theta_cos : Inport  Port=4
  Add : Sum  Inputs=+-
  Add1 : Sum
  Product{,1..3} (4 alike) : Product
  ualpha : Outport  OutDataTypeStr=single
  ubeta : Outport  Port=2  OutDataTypeStr=single
  wires:
  Product2/1 -> Add1/1
  Product/1 -> Add/1
  Add/1 -> ualpha/1
  Product3/1 -> Add1/2
  ud/1 -> Product/1, Product2/1
  theta_sin/1 -> Product1/2, Product2/2
  theta_cos/1 -> Product3/2, Product/2
  uq/1 -> Product1/1, Product3/1
  Product1/1 -> Add/2
  Add1/1 -> ubeta/1

== system positionloop/currloop1/Clark ==
  note: ialpha = ia*2/3-(ib+ic)/3;
      | ibeta = (ib-ic)*sqrt(3)/3;
  ia : Inport  OutDataTypeStr=single
  ib : Inport  Port=2  OutDataTypeStr=single
  ic : Inport  Port=3  OutDataTypeStr=single
  Add : Sum  OutDataTypeStr=single  AccumDataTypeStr=single
  Add1 : Sum  Inputs=+-  OutDataTypeStr=single  AccumDataTypeStr=single
  Add2 : Sum  Inputs=+-  OutDataTypeStr=single  AccumDataTypeStr=single
  Gain : Gain  Gain=2/3  ParamDataTypeStr=single
  Gain1 : Gain  Gain=1/3  ParamDataTypeStr=single
  Gain2 : Gain  Gain=sqrt(3)/3  ParamDataTypeStr=single
  ialpha : Outport  OutDataTypeStr=single
  ibeta : Outport  Port=2  OutDataTypeStr=single
  wires:
  Add1/1 -> ialpha/1
  ia/1 -> Gain/1
  Gain2/1 -> ibeta/1
  ib/1 -> Add/1, Add2/1
  Gain/1 -> Add1/1
  Add2/1 -> Gain2/1
  Add/1 -> Gain1/1
  ic/1 -> Add/2, Add2/2
  Gain1/1 -> Add1/2

== system positionloop/currloop1/Park ==
  note: id = ialpha*cos(theta)+ibeta*sin(theta);
      | iq = -ialpha*sin(theta)+ibeta*cos(theta);
  ialpha : Inport  OutDataTypeStr=single
  ibeta : Inport  Port=2  OutDataTypeStr=single
  theta_sin : Inport  Port=3  OutDataTypeStr=single
  theta_cos : Inport  Port=4  OutDataTypeStr=single
  Add : Sum  OutDataTypeStr=single  AccumDataTypeStr=single
  Add1 : Sum  Inputs=-+  OutDataTypeStr=single  AccumDataTypeStr=single
  Product{,1..3} (4 alike) : Product  OutDataTypeStr=single
  id : Outport  OutDataTypeStr=single
  iq : Outport  Port=2  OutDataTypeStr=single
  wires:
  theta_cos/1 -> Product/2, Product3/2
  ibeta/1 -> Product1/1, Product3/1
  Product1/1 -> Add/2
  Add1/1 -> iq/1
  Add/1 -> id/1
  Product3/1 -> Add1/2
  ialpha/1 -> Product/1, Product2/1
  Product2/1 -> Add1/1
  Product/1 -> Add/1
  theta_sin/1 -> Product1/2, Product2/2

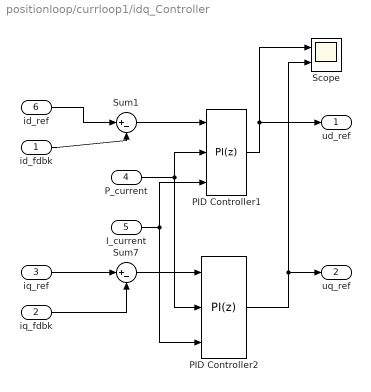
== system positionloop/currloop1/idq_Controller ==
  id_fdbk : Inport  OutDataTypeStr=single
  iq_fdbk : Inport  Port=2  OutDataTypeStr=single
  iq_ref : Inport  Port=3  OutDataTypeStr=single
  P_current : Inport  Port=4  OutDataTypeStr=single
  I_current : Inport  Port=5  OutDataTypeStr=single
  id_ref : Inport  Port=6  OutDataTypeStr=single
  PID Controller1 : slpidlib/PID Controller  Controller=PI  Form=Parallel  TimeDomain=Discrete-time  UseExternalTs=off  SampleTime=-1  IntegratorMethod=Forward Euler  FilterMethod=Forward Euler  ControllerParametersSource=external  P=curr_d_kp  I=curr_d_ki  UseKiTs=off  D=0  UseExternalDerivativeSource=off  N=100  UseFilter=on  TunerSelectOption=Transfer Function Based (PID Tuner App)  InitialConditionSource=internal  InitialConditionForIntegrator=0  InitialConditionForFilter=0  DifferentiatorICPrevScaledInput=0  ExternalReset=none  TrackingMode=off  Kt=1  LimitOutput=on  SatLimitsSource=internal  UpperSaturationLimit=48*0.9/sqrt(3)  LowerSaturationLimit=-48*0.9/sqrt(3)  LinearizeAsGain=on  AntiWindupMode=clamping  Kb=1  LimitIntegrator=off  UpperIntegratorSaturationLimit=inf  LowerIntegratorSaturationLimit=-inf  PGainOutDataTypeStr=single  PProdOutDataTypeStr=single  POutMin=[]  POutMax=[]  IGainOutDataTypeStr=int16  IProdOutDataTypeStr=int16  IOutMin=[]  IOutMax=[]  DOutMin=[]  DOutMax=[]  NOutMin=[]  NOutMax=[]  SumOutDataTypeStr=single  SumOutMin=[]  SumOutMax=[]  SaturationOutDataTypeStr=single  SaturationOutMin=[]  SaturationOutMax=[]  PParamMin=[]  PParamMax=[]  IParamMin=[]  IParamMax=[]  DParamMin=[]  DParamMax=[]  NParamMin=[]  NParamMax=[]  KbParamMin=[]  KbParamMax=[]  KtParamMin=[]  KtParamMax=[]  KbOutMin=[]  KbOutMax=[]  KtOutMin=[]  KtOutMax=[]  IntegratorOutMin=[]  IntegratorOutMax=[]  FilterOutMin=[]  FilterOutMax=[]  SumI1OutMin=[]  SumI1OutMax=[]  SumI2OutMin=[]  SumI2OutMax=[]  SumI3OutMin=[]  SumI3OutMax=[]  SumI4OutMin=[]  SumI4OutMax=[]  SumDOutMin=[]  SumDOutMax=[]  DifferentiatorOutMin=[]  DifferentiatorOutMax=[]  FilterDiffOutCoefMin=[]  FilterDiffOutCoefMax=[]  ReciprocalOutMin=[]  ReciprocalOutMax=[]  SumDenOutMin=[]  SumDenOutMax=[]  SumNumOutMin=[]  SumNumOutMax=[]  DivideOutMin=[]  DivideOutMax=[]  UdiffTsProdOutMin=[]  UdiffTsProdOutMax=[]  NTsProdOutMin=[]  NTsProdOutMax=[]  UintegralTsProdOutMin=[]  UintegralTsProdOutMax=[]  UngainTsProdOutMin=[]  UngainTsProdOutMax=[]  ClampingZeroOutDataTypeStr=Inherit: Inherit via back propagation  ClampingZeroOutMin=[]  ClampingZeroOutMax=[]  FilterDenConstantOutDataTypeStr=Inherit: Inherit via back propagation  FilterDenConstantOutMin=[]  FilterDenConstantOutMax=[]  PCopyOutDataTypeStr=Inherit: Inherit via back propagation  PCopyOutMin=[]  PCopyOutMax=[]  NCopyOutDataTypeStr=Inherit: Inherit via back propagation  NCopyOutMin=[]  NCopyOutMax=[]  IntegratorContinuousStateAttributes=''  IntegratorStateMustResolveToSignalObject=off  IntegratorRTWStateStorageClass=Auto  FilterContinuousStateAttributes=''  FilterStateMustResolveToSignalObject=off  FilterRTWStateStorageClass=Auto  ParallelPVariant=ExternalParameters  IdealPVariant=Disabled  IVariant=ExternalParameters  DVariant=Disabled  IntegratorVariant=Discrete  SatVariant=Enabled  AWVariant=DiscClampingParallel  PCopyVariant=Disabled  TRVariant=Disabled  FdbkBlocksVariant=Forward  IdealPFdbkVariant=Disabled  SatFdbkVariant=Disabled  DerivativeFilterVariant=Disabled  NVariant=Disabled  NCopyVariant=Disabled_SignalSpec  FilterICVariant=Disabled  IntegratorICVariant=InternalICs  ExternalResetVariant=Disabled  TRSumVariant=Passthrough  SumFdbkVariant=Disabled  SumVariant=Sum_PI  TsampFilterVariant=InternalTs  TsampNgainVariant=Passthrough  TsampIntegralVariant=Disabled_SignalSpec  ExternalSaturationOutDataTypeStr=Inherit: Same as second input  DerivativeSourceVariant=Disabled
  PID Controller2 : slpidlib/PID Controller  Controller=PI  Form=Parallel  TimeDomain=Discrete-time  UseExternalTs=off  SampleTime=-1  IntegratorMethod=Forward Euler  FilterMethod=Forward Euler  ControllerParametersSource=external  P=curr_q_kp  I=curr_q_ki  UseKiTs=off  D=0  UseExternalDerivativeSource=off  N=100  UseFilter=on  TunerSelectOption=Transfer Function Based (PID Tuner App)  InitialConditionSource=internal  InitialConditionForIntegrator=0  InitialConditionForFilter=0  DifferentiatorICPrevScaledInput=0  ExternalReset=none  TrackingMode=off  Kt=1  LimitOutput=on  SatLimitsSource=internal  UpperSaturationLimit=48*0.9/sqrt(3)  LowerSaturationLimit=-48*0.9/sqrt(3)  LinearizeAsGain=on  AntiWindupMode=clamping  Kb=1  LimitIntegrator=off  UpperIntegratorSaturationLimit=inf  LowerIntegratorSaturationLimit=-inf  PGainOutDataTypeStr=single  PProdOutDataTypeStr=single  POutMin=[]  POutMax=[]  IGainOutDataTypeStr=single  IProdOutDataTypeStr=single  IOutMin=[]  IOutMax=[]  DOutMin=[]  DOutMax=[]  NOutMin=[]  NOutMax=[]  SumOutDataTypeStr=single  SumOutMin=[]  SumOutMax=[]  SaturationOutDataTypeStr=single  SaturationOutMin=[]  SaturationOutMax=[]  PParamMin=[]  PParamMax=[]  IParamMin=[]  IParamMax=[]  DParamMin=[]  DParamMax=[]  NParamMin=[]  NParamMax=[]  KbParamMin=[]  KbParamMax=[]  KtParamMin=[]  KtParamMax=[]  KbOutMin=[]  KbOutMax=[]  KtOutMin=[]  KtOutMax=[]  IntegratorOutMin=[]  IntegratorOutMax=[]  FilterOutMin=[]  FilterOutMax=[]  SumI1OutMin=[]  SumI1OutMax=[]  SumI2OutMin=[]  SumI2OutMax=[]  SumI3OutMin=[]  SumI3OutMax=[]  SumI4OutMin=[]  SumI4OutMax=[]  SumDOutMin=[]  SumDOutMax=[]  DifferentiatorOutMin=[]  DifferentiatorOutMax=[]  FilterDiffOutCoefMin=[]  FilterDiffOutCoefMax=[]  ReciprocalOutMin=[]  ReciprocalOutMax=[]  SumDenOutMin=[]  SumDenOutMax=[]  SumNumOutMin=[]  SumNumOutMax=[]  DivideOutMin=[]  DivideOutMax=[]  UdiffTsProdOutMin=[]  UdiffTsProdOutMax=[]  NTsProdOutMin=[]  NTsProdOutMax=[]  UintegralTsProdOutMin=[]  UintegralTsProdOutMax=[]  UngainTsProdOutMin=[]  UngainTsProdOutMax=[]  ClampingZeroOutDataTypeStr=Inherit: Inherit via back propagation  ClampingZeroOutMin=[]  ClampingZeroOutMax=[]  FilterDenConstantOutDataTypeStr=Inherit: Inherit via back propagation  FilterDenConstantOutMin=[]  FilterDenConstantOutMax=[]  PCopyOutDataTypeStr=Inherit: Inherit via back propagation  PCopyOutMin=[]  PCopyOutMax=[]  NCopyOutDataTypeStr=Inherit: Inherit via back propagation  NCopyOutMin=[]  NCopyOutMax=[]  IntegratorContinuousStateAttributes=''  IntegratorStateMustResolveToSignalObject=off  IntegratorRTWStateStorageClass=Auto  FilterContinuousStateAttributes=''  FilterStateMustResolveToSignalObject=off  FilterRTWStateStorageClass=Auto  ParallelPVariant=ExternalParameters  IdealPVariant=Disabled  IVariant=ExternalParameters  DVariant=Disabled  IntegratorVariant=Discrete  SatVariant=Enabled  AWVariant=DiscClampingParallel  PCopyVariant=Disabled  TRVariant=Disabled  FdbkBlocksVariant=Forward  IdealPFdbkVariant=Disabled  SatFdbkVariant=Disabled  DerivativeFilterVariant=Disabled  NVariant=Disabled  NCopyVariant=Disabled_SignalSpec  FilterICVariant=Disabled  IntegratorICVariant=InternalICs  ExternalResetVariant=Disabled  TRSumVariant=Passthrough  SumFdbkVariant=Disabled  SumVariant=Sum_PI  TsampFilterVariant=InternalTs  TsampNgainVariant=Passthrough  TsampIntegralVariant=Disabled_SignalSpec  ExternalSaturationOutDataTypeStr=Inherit: Same as second input  DerivativeSourceVariant=Disabled
  Scope : Scope  NumInputPorts=2
  Sum1 : Sum  Inputs=|+-  OutDataTypeStr=single  AccumDataTypeStr=single
  Sum7 : Sum  Inputs=|+-  OutDataTypeStr=single  AccumDataTypeStr=single
  ud_ref : Outport  OutDataTypeStr=single
  uq_ref : Outport  Port=2  OutDataTypeStr=single
  wires:
  id_fdbk/1 -> Sum1/2
  id_ref/1 -> Sum1/1
  iq_fdbk/1 -> Sum7/2
  Sum1/1 -> PID Controller1/1
  Sum7/1 -> PID Controller2/1
  PID Controller1/1 -> Scope/1, ud_ref/1
  PID Controller2/1 -> Scope/2, uq_ref/1
  iq_ref/1 -> Sum7/1
  P_current/1 -> PID Controller2/2, PID Controller1/2
  I_current/1 -> PID Controller2/3, PID Controller1/3

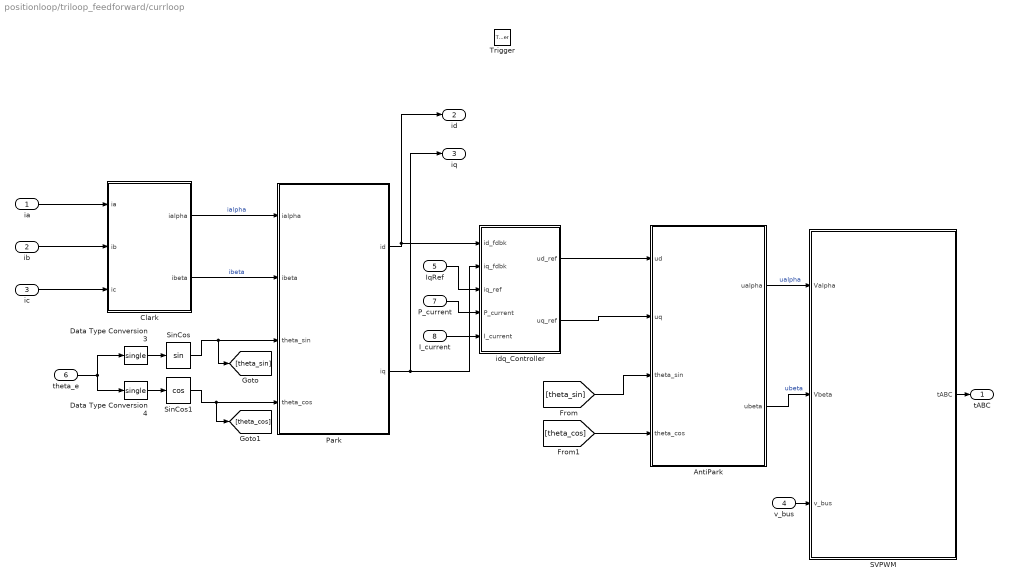
== system positionloop/triloop_feedforward/currloop ==
  ia : Inport
  ib : Inport  Port=2
  ic : Inport  Port=3
  v_bus : Inport  Port=4
  IqRef : Inport  Port=5
  theta_e : Inport  Port=6
  P_current : Inport  Port=7
  I_current : Inport  Port=8
  Trigger : TriggerPort  TriggerType=function-call  VariantControl=(inherit)  PortDimensions=1
  AntiPark : Subsystem
  Clark : Subsystem
  Data Type Conversion3 : DataTypeConversion  OutDataTypeStr=single  SaturateOnIntegerOverflow=off  RndMeth=Floor
  Data Type Conversion4 : DataTypeConversion  OutDataTypeStr=single  SaturateOnIntegerOverflow=off  RndMeth=Floor
  Park : Subsystem
  SVPWM : Subsystem  TreatAsAtomicUnit=on
  SinCos : Trigonometry
  SinCos1 : Trigonometry  Operator=cos
  idq_Controller : Subsystem
  tABC : Outport
  id : Outport  Port=2
  iq : Outport  Port=3
  wires:
  Data Type Conversion4/1 -> SinCos1/1
  Data Type Conversion3/1 -> SinCos/1
  AntiPark/2(ubeta) -> SVPWM/2(Vbeta)  "ubeta"
  AntiPark/1(ualpha) -> SVPWM/1(Valpha)  "ualpha"
  [theta_cos] -> AntiPark/4(theta_cos)
  [theta_sin] -> AntiPark/3(theta_sin)
  SinCos/1 -> Park/3(theta_sin), [theta_sin]
  theta_e/1 -> Data Type Conversion3/1, Data Type Conversion4/1
  SinCos1/1 -> Park/4(theta_cos), [theta_cos]
  v_bus/1 -> SVPWM/3(v_bus)
  SVPWM/1(tABC) -> tABC/1
  ib/1 -> Clark/2(ib)
  ia/1 -> Clark/1(ia)
  ic/1 -> Clark/3(ic)
  Clark/1(ialpha) -> Park/1(ialpha)  "ialpha"
  Clark/2(ibeta) -> Park/2(ibeta)  "ibeta"
  idq_Controller/1(ud_ref) -> AntiPark/1(ud)
  idq_Controller/2(uq_ref) -> AntiPark/2(uq)
  Park/1(id) -> id/1, idq_Controller/1(id_fdbk)
  Park/2(iq) -> iq/1, idq_Controller/2(iq_fdbk)
  IqRef/1 -> idq_Controller/3(iq_ref)
  I_current/1 -> idq_Controller/5(I_current)
  P_current/1 -> idq_Controller/4(P_current)

== system positionloop/triloop_feedforward/positionloop ==
  PositionRef : Inport
  PositionFd : Inport  Port=2
  P_position : Inport  Port=3
  Trigger : TriggerPort  TriggerType=function-call  VariantControl=(inherit)  PortDimensions=1
  Subsystem : Subsystem
  SpeedRef : Outport
  wires:
  PositionRef/1 -> Subsystem/1(PositionRef)
  PositionFd/1 -> Subsystem/2(PositionFd)
  Subsystem/1(SpeedRef) -> SpeedRef/1
  P_position/1 -> Subsystem/3(P_position)

== system positionloop/triloop_feedforward/speedloop ==
  SpeedRef : Inport
  SpeedFd : Inport  Port=2
  P_speed : Inport  Port=3
  I_speed : Inport  Port=4
  Trigger : TriggerPort  TriggerType=function-call  VariantControl=(inherit)  PortDimensions=1
  Subsystem : Subsystem
  iqRef : Outport
  wires:
  SpeedRef/1 -> Subsystem/1(SpeedRef)
  SpeedFd/1 -> Subsystem/2(SpeedFd)
  Subsystem/1(iqRef) -> iqRef/1
  P_speed/1 -> Subsystem/3(P_speed)
  I_speed/1 -> Subsystem/4(I_speed)

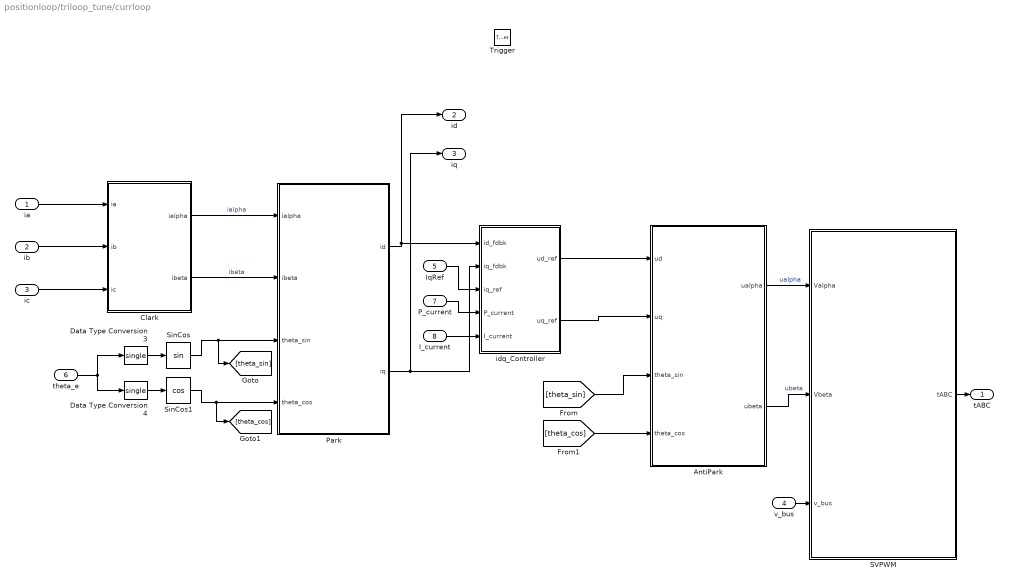
== system positionloop/triloop_tune/currloop ==
  ia : Inport
  ib : Inport  Port=2
  ic : Inport  Port=3
  v_bus : Inport  Port=4
  IqRef : Inport  Port=5
  theta_e : Inport  Port=6
  P_current : Inport  Port=7
  I_current : Inport  Port=8
  Trigger : TriggerPort  TriggerType=function-call  VariantControl=(inherit)  PortDimensions=1
  AntiPark : Subsystem
  Clark : Subsystem
  Data Type Conversion3 : DataTypeConversion  OutDataTypeStr=single  SaturateOnIntegerOverflow=off  RndMeth=Floor
  Data Type Conversion4 : DataTypeConversion  OutDataTypeStr=single  SaturateOnIntegerOverflow=off  RndMeth=Floor
  Park : Subsystem
  SVPWM : Subsystem  TreatAsAtomicUnit=on
  SinCos : Trigonometry
  SinCos1 : Trigonometry  Operator=cos
  idq_Controller : Subsystem
  tABC : Outport
  id : Outport  Port=2
  iq : Outport  Port=3
  wires:
  Data Type Conversion4/1 -> SinCos1/1
  Data Type Conversion3/1 -> SinCos/1
  AntiPark/2(ubeta) -> SVPWM/2(Vbeta)  "ubeta"
  AntiPark/1(ualpha) -> SVPWM/1(Valpha)  "ualpha"
  [theta_cos] -> AntiPark/4(theta_cos)
  [theta_sin] -> AntiPark/3(theta_sin)
  SinCos/1 -> Park/3(theta_sin), [theta_sin]
  theta_e/1 -> Data Type Conversion3/1, Data Type Conversion4/1
  SinCos1/1 -> Park/4(theta_cos), [theta_cos]
  v_bus/1 -> SVPWM/3(v_bus)
  SVPWM/1(tABC) -> tABC/1
  ib/1 -> Clark/2(ib)
  ia/1 -> Clark/1(ia)
  ic/1 -> Clark/3(ic)
  Clark/1(ialpha) -> Park/1(ialpha)  "ialpha"
  Clark/2(ibeta) -> Park/2(ibeta)  "ibeta"
  idq_Controller/1(ud_ref) -> AntiPark/1(ud)
  idq_Controller/2(uq_ref) -> AntiPark/2(uq)
  Park/1(id) -> id/1, idq_Controller/1(id_fdbk)
  Park/2(iq) -> iq/1, idq_Controller/2(iq_fdbk)
  IqRef/1 -> idq_Controller/3(iq_ref)
  I_current/1 -> idq_Controller/5(I_current)
  P_current/1 -> idq_Controller/4(P_current)

== system positionloop/triloop_tune/positionloop ==
  PositionRef : Inport
  PositionFd : Inport  Port=2
  P_position : Inport  Port=3
  Trigger : TriggerPort  TriggerType=function-call  VariantControl=(inherit)  PortDimensions=1
  Subsystem : Subsystem
  SpeedRef : Outport
  wires:
  PositionRef/1 -> Subsystem/1(PositionRef)
  PositionFd/1 -> Subsystem/2(PositionFd)
  Subsystem/1(SpeedRef) -> SpeedRef/1
  P_position/1 -> Subsystem/3(P_position)

== system positionloop/triloop_tune/speedloop ==
  SpeedRef : Inport
  SpeedFd : Inport  Port=2
  P_speed : Inport  Port=3
  I_speed : Inport  Port=4
  Trigger : TriggerPort  TriggerType=function-call  VariantControl=(inherit)  PortDimensions=1
  Subsystem : Subsystem
  iqRef : Outport
  wires:
  SpeedRef/1 -> Subsystem/1(SpeedRef)
  SpeedFd/1 -> Subsystem/2(SpeedFd)
  Subsystem/1(iqRef) -> iqRef/1
  P_speed/1 -> Subsystem/3(P_speed)
  I_speed/1 -> Subsystem/4(I_speed)

== system positionloop/currloop/SVPWM/AntiClark ==
  note: Va = Valpha;
      | Vb = Valpha*(-1/2)+Vbeta*sqrt(3)/3
      | Vc = Valpha*(-1/2)-Vbeta*sqrt(3)/3
  Valpha : Inport  OutDataTypeStr=single
  Vbeta : Inport  Port=2  OutDataTypeStr=single
  Gain : Gain  Gain=-1/2  OutDataTypeStr=single
  Gain1 : Gain  Gain=sqrt(3)/2  OutDataTypeStr=single
  Sum : Sum  Inputs=|++  OutDataTypeStr=single
  Sum1 : Sum  Inputs=-+|  OutDataTypeStr=single
  Va : Outport  OutDataTypeStr=single
  Vb : Outport  Port=2  OutDataTypeStr=single
  Vc : Outport  Port=3  OutDataTypeStr=single
  wires:
  Sum1/1 -> Vc/1
  Gain1/1 -> Sum1/1, Sum/2
  Sum/1 -> Vb/1
  Gain/1 -> Sum/1, Sum1/2
  Vbeta/1 -> Gain1/1
  Valpha/1 -> Va/1, Gain/1
